simulink model "follow"  (R2024a)
settings: Solver=VariableStepAuto  StartTime=0.0  StopTime=10.0  RelTol=1e-5
values from neighbouring files (symbols this model uses):
  A = [0, 1, 0, 0 ... (first row only)    [get_matrices.m]    (also in main.m)
  B = [0; 4 / (4 * M + m); 0; 3 / (l * (4 * M + m))]    [get_matrices.m]    (also in main.m = [0; 0; 1 / M; -1 / (l * M)])
  C = [1, 0, 0, 0; 0, 0, 1, 0]    [get_matrices.m]    (also in main.m)
  D = [0; 3 / (l * (4 * M + m)); 0; 3 * (M + m) / ((m * l * l) * (4 * M + m))]    [get_matrices.m]    (also in main.m = [0; -1/(l * M); 0; (M + m) / (m * l * l * M)])
  Gamma_f = [0 -1 0 0 0 0 0 0 0 0 ... (first row only)    [chapter5.m]
  K = -R \ B' * P    [TAU.m]    (also in chapter3.m = TAU.FindControllerSylvester(A, B, GammaK); chapter4.m = pairs{i}{1}; chapter6.m = TAU.FindControllerLMI(A, B, 2); main.m = FindControllerSylvester(A, B, Gamma))
  Kf = GetFollowController(A, B, Gamma_f, Y_f, Cz, K)    [chapter5.m]
  l = l / 2    [get_initials.m]    (also in main.m)
  M = randi([100000 1000000]) / 1000 / sqrt(2)    [get_initials.m]    (also in main.m)
  m = randi([1000 10000]) / 1000 * sqrt(3)    [get_initials.m]    (also in main.m)
  theta0 = 0.1    [chapter2.m]    (also in chapter3.m; chapter4.m = 0.2; chapter5.m = 0.2; chapter6.m = 0.2)
  w0 = [1.0, 0, 0, 0, 0.3, 0, 0, 0, 0.5, 0]'    [chapter5.m]
  Y_f = [0.3, -0.5, 0.2, -1, 0.9, 0.4, 0.6, 0.8, -0.7, 0.1]    [chapter5.m]
settings Model: Creator=alexivanov  LastModifiedBy=alexivanov

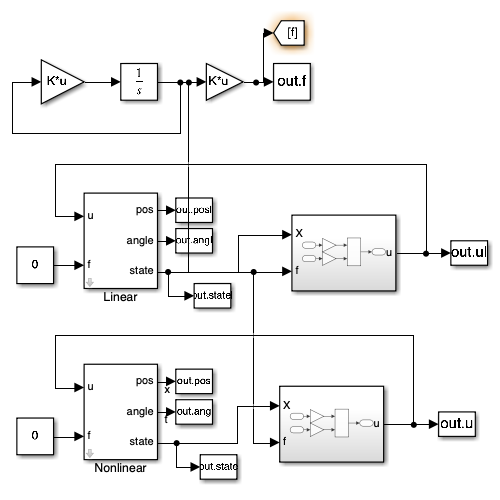
[thumbnail: Simulink's stored preview of the top-level diagram]
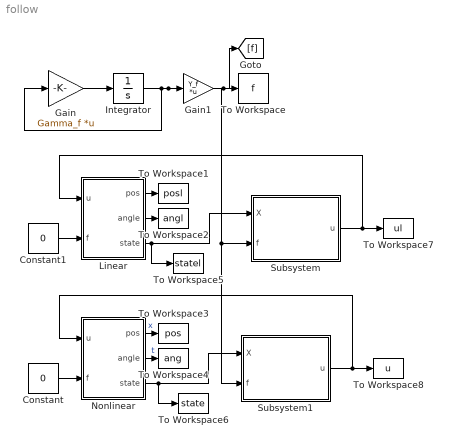
== system follow ==
  Constant : Constant  Value=0
  Constant1 : Constant  Value=0
  Gain : Gain  Gain=Gamma_f  Multiplication=Matrix(K*u)
  Gain1 : Gain  Gain=Y_f  Multiplication=Matrix(K*u)
  Integrator : Integrator  InitialCondition=w0
  Linear : Subsystem  mask{Mcart=M, m=m, l=l, g=9.81, theta0=theta0}
      mask prompts: Mcart "Mass of cart (kg)"; m "Mass of pend (kg)"; l "Length of pend (m)"; theta0 "Initial angle (rad)"
  Nonlinear : Subsystem  mask{Mcart=M, m=m, l=l, g=9.81, theta0=theta0}
      mask prompts: Mcart "Mass of cart (kg)"; m "Mass of pend (kg)"; l "Length of pend (m)"; theta0 "Initial angle (rad)"
  Subsystem : Subsystem
  Subsystem1 : Subsystem
  To Workspace : ToWorkspace  VariableName=f  SampleTime=-1
  To Workspace1 : ToWorkspace  VariableName=posl  SampleTime=-1
  To Workspace2 : ToWorkspace  VariableName=angl  SampleTime=-1
  To Workspace3 : ToWorkspace  VariableName=pos  SampleTime=-1
  To Workspace4 : ToWorkspace  VariableName=ang  SampleTime=-1
  To Workspace5 : ToWorkspace  VariableName=statel  SampleTime=-1
  To Workspace6 : ToWorkspace  VariableName=state  SampleTime=-1
  To Workspace7 : ToWorkspace  VariableName=ul  SampleTime=-1
  To Workspace8 : ToWorkspace  VariableName=u  SampleTime=-1
  wires:
  Subsystem1/1(u) -> To Workspace8/1, Nonlinear/1(u)
  Nonlinear/3(state) -> To Workspace6/1, Subsystem1/1(X)
  Constant1/1 -> Linear/2(f)
  Constant/1 -> Nonlinear/2(f)
  Gain1/1 -> [f], To Workspace/1
  Integrator/1 -> Gain/1, Subsystem1/2(f), Subsystem/2(f), Gain1/1
  Nonlinear/2(angle) -> To Workspace4/1  "t"
  Linear/1(pos) -> To Workspace1/1
  Gain/1 -> Integrator/1
  Nonlinear/1(pos) -> To Workspace3/1  "x"
  Subsystem/1(u) -> To Workspace7/1, Linear/1(u)
  Linear/3(state) -> To Workspace5/1, Subsystem/1(X)
  Linear/2(angle) -> To Workspace2/1

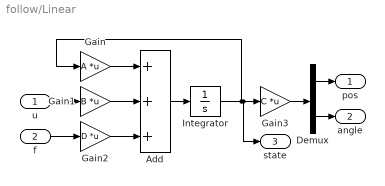
== system follow/Linear ==
  u : Inport
  f : Inport  Port=2
  Add : Sum  Inputs=+++
  Demux : Demux  Outputs=2
  Gain : Gain  Gain=A  Multiplication=Matrix(K*u)
  Gain1 : Gain  Gain=B  Multiplication=Matrix(K*u)
  Gain2 : Gain  Gain=D  Multiplication=Matrix(K*u)
  Gain3 : Gain  Gain=C  Multiplication=Matrix(K*u)
  Integrator : Integrator  InitialCondition=[0; 0; theta0; 0]
  pos : Outport
  angle : Outport  Port=2
  state : Outport  Port=3
  wires:
  Integrator/1 -> state/1, Gain3/1, Gain/1
  f/1 -> Gain2/1
  Gain3/1 -> Demux/1
  Add/1 -> Integrator/1
  Demux/1 -> pos/1
  Demux/2 -> angle/1
  Gain2/1 -> Add/3
  u/1 -> Gain1/1
  Gain/1 -> Add/1
  Gain1/1 -> Add/2

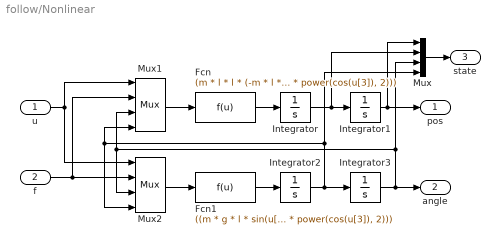
== system follow/Nonlinear ==
  u : Inport
  f : Inport  Port=2
  Fcn : Fcn  Expr=(m * l * l * (-m * l * power(u[4], 2) * sin(u[3]) + u[1]) + m * l * cos(u[3]) * (m * g * l * sin(u[3]) + u[2])) / (m * l * l * (Mcart + m - m * power(cos(u[3]), 2)))
  Fcn1 : Fcn  Expr=((m * g * l * sin(u[3]) + u[2]) * (Mcart + m) + m * l * cos(u[3]) * (-m * l * power(u[4], 2) * sin(u[3]) + u[1])) / (m * l * l * (Mcart + m - m * power(cos(u[3]), 2)))
  Integrator : Integrator
  Integrator1 : Integrator
  Integrator2 : Integrator
  Integrator3 : Integrator  InitialCondition=theta0
  Mux : Mux
  Mux1 : Mux
  Mux2 : Mux
  pos : Outport
  angle : Outport  Port=2
  state : Outport  Port=3
  wires:
  Integrator1/1 -> Mux/1, pos/1
  Integrator/1 -> Mux/2, Integrator1/1
  Integrator2/1 -> Mux/4, Mux1/4, Mux2/4, Integrator3/1
  Integrator3/1 -> Mux/3, Mux2/3, Mux1/3, angle/1
  Fcn/1 -> Integrator/1
  u/1 -> Mux2/1, Mux1/1
  f/1 -> Mux2/2, Mux1/2
  Fcn1/1 -> Integrator2/1
  Mux2/1 -> Fcn1/1
  Mux1/1 -> Fcn/1
  Mux/1 -> state/1

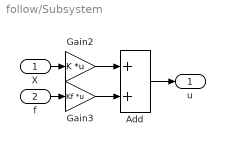
== system follow/Subsystem ==
  X : Inport
  f : Inport  Port=2
  Add : Sum
  Gain2 : Gain  Gain=K  Multiplication=Matrix(K*u)
  Gain3 : Gain  Gain=Kf  Multiplication=Matrix(K*u)
  u : Outport
  wires:
  Gain3/1 -> Add/2
  Gain2/1 -> Add/1
  X/1 -> Gain2/1
  Add/1 -> u/1
  f/1 -> Gain3/1

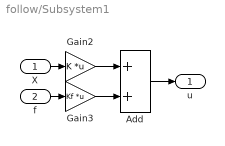
== system follow/Subsystem1 ==
  X : Inport
  f : Inport  Port=2
  Add : Sum
  Gain2 : Gain  Gain=K  Multiplication=Matrix(K*u)
  Gain3 : Gain  Gain=Kf  Multiplication=Matrix(K*u)
  u : Outport
  wires:
  Gain3/1 -> Add/2
  Gain2/1 -> Add/1
  X/1 -> Gain2/1
  Add/1 -> u/1
  f/1 -> Gain3/1
